simulink model "open_loop_system"  (Simulink 7.9)
settings: Solver=ode45  StartTime=0.0  StopTime=10.0  RelTol=1e-3
libraries: powerlib x4, powerlib_extras x1
settings Model: Creator=storm  LastModifiedBy=storm

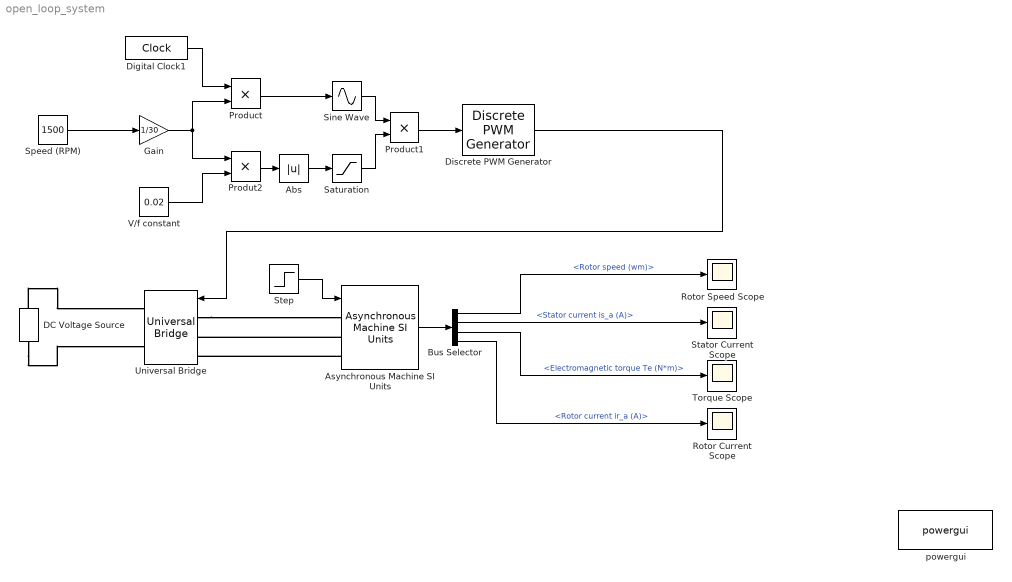
== system open_loop_system ==
  Abs : Abs
  Asynchronous Machine SI Units : powerlib/Machines/Asynchronous Machine SI Units  PresetModel=No  MechanicalLoad=Torque Tm  ShowDetailedParameters=on  RotorType=Squirrel-cage  ReferenceFrame=Rotor  NominalParameters=[ 120, 220, 50 ]  Stator=[22.143 0.18451]  Rotor=[ 14.3764 0.18451]  Cage1=[ 0.022 0.226/377]  Cage2=[ 0.022 0.226/377]  Lm=1  Mechanical="[ 0.0005 0  2 ]"  PolePairs=2  InitialConditions=[1 0 0 0 0 0 0 0]  Units=SI  LoadFlowParameters=1492000  SimulateSaturation=off  Saturation=[14.03593122, 27.81365428, 53.79336849, 72.68890987, 97.98006896, 148.6815601, 215.7428561, 302.9841135, 420.4778367 ; 230, 322, 414, 460, 506, 552, 598, 644, 690]  TsPowergui=0  TsBlock=-1  IterativeModel=Forward Euler  Pmec=0
  Bus Selector : BusSelector  OutputSignals=Mechanical.Rotor speed (wm),Stator measurements.Stator current is_a (A),Mechanical.Electromagnetic torque Te (N*m),Rotor measurements.Rotor current ir_a (A)
  DC Voltage Source : powerlib/Electrical Sources/DC Voltage Source  Amplitude=270  Measurements=None
  Digital Clock1 : DigitalClock  SampleTime=5e-05
  Discrete PWM Generator : powerlib_extras/Discrete  Control Blocks/Discrete PWM Generator  GeneratorMode="3-arm  bridge (6 pulses)"  Fc=12000  Ts=5e-05  Internal=off  mIndex=1  Freq=50  Phase=0
  Gain : Gain  Gain=1/30
  Product : Product  RndMeth=Zero
  Product1 : Product  RndMeth=Zero
  Produt2 : Product  RndMeth=Zero
  Rotor Current Scope : Scope
      settings: TimeRange=10  YMin=-0.35  YMax=0.3  SaveName=ScopeData2
  Rotor Speed Scope : Scope
      settings: TimeRange=10  YMin=20  YMax=170
  Saturation : Saturate  UpperLimit=1  LowerLimit=0.1
  Sine Wave : Sin  TimeSource=Use external signal  Frequency=2*pi  Phase=[0 240*(pi/180) 120*(pi/180)]  SampleTime=0
  Speed (RPM) : Constant  Value=1500
  Stator Current Scope : Scope
      settings: TimeRange=10  YMin=-0.7  YMax=0.7  SaveName=ScopeData4
  Step : Step  Time=2  After=0.4  SampleTime=0
  Torque Scope : Scope
      settings: TimeRange=10  YMin=-0.1  YMax=0.55
  Universal Bridge : powerlib/Power Electronics/Universal Bridge  Arms=3  SnubberResistance=1e5  SnubberCapacitance=inf  Device=MOSFET / Diodes  Ron=1e-3  Lon=0  ForwardVoltages="[  0  0  ]"  ForwardVoltage=0  GTOparameters=[ 10e-6 , 20e-6 ]  IGBTparameters=[ 1e-6 , 2e-6 ]  Measurements=None  Measurements_2=None  converterType=Rectifier
  V/f constant : Constant  Value=0.02
  powergui : powerlib/powergui  Priority=1  SimulationMode=Discrete  SolverType=Tustin  SampleTime=50e-6  frequency=60  SPID=off  DisableSnubberDevices=off  DisableRonSwitches=off  DisableVfSwitches=off  SwTol=0  Interpol=off  DisplayEquations=off  FunctionMessages=off  frequencyindice=50  Pbase=100e6  ErrMax=1e-4  Iterations=50  UnitsV=kV  UnitsW=MW  echomessages=off  HookPort=off  EnableUseOfTLC=off  x0status=blocks  RestoreLinks=warning  ResistiveCurrentMeasurement=off  Ylog=off  Xlog=on  ShowGrid=off  save=off  variable=ZData  ZoomFFT=off  StartTime=0.0  cycles=1  DisplayStyle=1  FreqAxis=off  MaxFrequency=1000  frequencyindicesteady=1  display=off  methode=off
  wires:
  Asynchronous Machine SI Units/1 -> Bus Selector/1
  Bus Selector/1 -> Rotor Speed Scope/1  "<Rotor speed (wm)>"
  Step/1 -> Asynchronous Machine SI Units/1
  Discrete PWM Generator/1 -> Universal Bridge/1
  Bus Selector/2 -> Stator Current Scope/1  "<Stator current is_a (A)>"
  Product/1 -> Sine Wave/1
  Digital Clock1/1 -> Product/1
  Sine Wave/1 -> Product1/1
  Saturation/1 -> Product1/2
  Produt2/1 -> Abs/1
  V/f constant/1 -> Produt2/2
  Abs/1 -> Saturation/1
  Product1/1 -> Discrete PWM Generator/1
  Speed (RPM)/1 -> Gain/1
  Gain/1 -> Product/2, Produt2/1
  Bus Selector/3 -> Torque Scope/1  "<Electromagnetic torque Te (N*m)>"
  Bus Selector/4 -> Rotor Current Scope/1  "<Rotor current ir_a (A)>"
  connections:
  DC Voltage Source/LConn1 -- Universal Bridge/RConn2
  DC Voltage Source/RConn1 -- Universal Bridge/RConn1
  Asynchronous Machine SI Units/LConn3 -- Universal Bridge/LConn3
  Universal Bridge/LConn1 -- Asynchronous Machine SI Units/LConn1
  Asynchronous Machine SI Units/LConn2 -- Universal Bridge/LConn2
